simulink model "doc_scalar_quant_2"  (Simulink 5.0)
settings: Solver=ode45  StartTime=0.0  StopTime=2*pi  RelTol=1e-3
undefined symbols (not defined in the file): slcm
libraries: commsrccod2 x1
settings Model: Creator=agaltman  LastModifiedBy=agaltman  SignalLoggingName=logsOut  BlockReductionOpt=off  BooleanDataType=off  ConditionalExecOptimization=on  ZeroCrossControl=UseLocalSettings  RTWMathFcnLibMatFile=iso_c_tmw.mat  RTWOptions="-aEnforceIntegerDowncast=1 -aFoldNonRolledExpr=1 -aInlineInvariantSignals=1 -aInlineParameters=0 -aLocalBlockOutputs=1 -aRollThreshold=5 -aRTWVerbose=1 -aGenerateReport=0 -aForceParamTrailComments=0 -aGenerateComments=1 -aIgnoreCustomStorageClasses=1 -aIncHierarchyInIds=0 -aMaxRTWIdLen=31 -aShowEliminatedStatements=0 -aReadOnly=0 -aIncDataTypeInIds=0 -aPrefixModelToSubsysFcnNames=1 -aInlinedPrmAccess=\"Literals\" -aGenerateFullHeader=1 -aIsPILTarget=0 -aLogVarNameModifier=\"rt_\" -aExtMode=0 -aExtModeTesting=0 -aExtModeTransport=\"tcpip\""

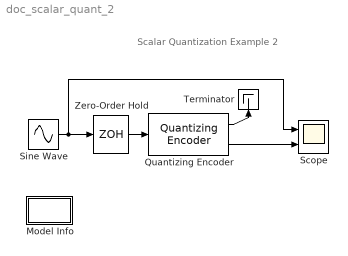
== system doc_scalar_quant_2 ==
  note: Scalar Quantization Example 2
  Model Info : Subsystem  LoadFcn=slcm LoadBlock;  InitFcn=slcm('UpdateAllCMBlocksInThisModelInit')  mask(CMBlock){InitialSaveTempField=, InitialBlockCM=none, BlockCM=none, Frame=on, SaveTempField=, DisplayStringWithTags=Info, MaskDisplayString=Info, HorizontalTextAlignment=Center, LeftAlignmentValue=0.5, SourceBlockDiagram=doc_scalar_quant_2, TagMaxNumber=20, CMTag1=, CMTag2=, CMTag3=, CMTag4=, CMTag5=, CMTag6=, CMTag7=, CMTag8=, CMTag9=, CMTag10=, CMTag11=, CMTag12=, CMTag13=, CMTag14=, CMTag15=, CMTag16=, CMTag17=, CMTag18=, CMTag19=, CMTag20=}
      mask help: This block allows revision control information to be displayed within the model.
      settings: CopyFcn=slcm CopyBlock;  DeleteFcn=slcm Cancel;  PostSaveFcn=slcm('UpdateAllCMBlocksInThisModel')  NameChangeFcn=slcm Rename;  OpenFcn=commdemohelp;
      mask Display: text(str2num(LeftAlignmentValue), 0.5, MaskDisplayString, 'HorizontalAlignment', HorizontalTextAlignment)
  Quantizing Encoder : commsrccod2/Quantizing Encoder  partition=[-1:.2:1]  codebook=[-1.1:.2:1.1]
  Scope : Scope  NumInputPorts=2
      settings: YMin=-1.2~-1.2  YMax=1.2~1.2
  Sine Wave : Sin  SampleTime=0
  Terminator : Terminator
      settings: Orientation=up
  Zero-Order Hold : ZeroOrderHold  SampleTime=.1
  wires:
  Quantizing Encoder/1 -> Terminator/1
  Quantizing Encoder/2 -> Scope/2
  Sine Wave/1 -> Scope/1, Zero-Order Hold/1
  Zero-Order Hold/1 -> Quantizing Encoder/1

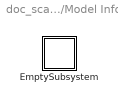
== system doc_scalar_quant_2/Model Info ==
  EmptySubsystem : Subsystem

== system doc_scalar_quant_2/Model Info/EmptySubsystem ==
